simulink model "SP_OEL2"  (R2023b)
settings: Solver=ode23t  StartTime=0.0  StopTime=0.6  MaxStep=simulation.maxStepSize  RelTol=1e-3  AbsTol=1e-3
PostLoadFcn:
  | run('OCR_input.m');
  | run('OCR_settings.m');
InitFcn:
  | run('OCR_settings.m');
undefined symbols (not defined in the file or in its folder): relay1, relay2, source
libraries: ee_lib x14, fl_lib x8, eeGeneralControl x8, simulink x4, simulink_extras x4, nesl_utility x2
(part 2 of 2)

== system SP_OEL2/Relay1/Phase Protection Unit/Operating time /Lookup table  ==
  Current : Inport
  2-D Lookup Table : Lookup_n-D  BreakpointsForDimension1=currentPhase  BreakpointsForDimension2=tmsPhase  Table=topPhase  InterpMethod=Cubic spline  ExtrapMethod=Cubic spline  InternalRulePriority=Speed  RndMeth=Simplest
      settings: InputPortMap=u0,u1
  Constant12 : Constant  Value=phTimeSetting  VectorParams1D=off
  Constant14 : Constant  Value=topPhaseActual
  Constant15 : Constant  Value=relayCharacteristicPhase
  Demux2 : Demux  Outputs=3
  Max : MinMax  Function=max  Inputs=3
  Switch3 : Switch  Threshold=8  SaturateOnIntegerOverflow=off  InputSameDT=off
  Operating Time : Outport
  wires:
  Constant15/1 -> Switch3/2
  Current/1 -> Demux2/1
  Constant12/1 -> 2-D Lookup Table/2
  Demux2/2 -> Max/2
  Demux2/1 -> Max/1
  Constant14/1 -> Switch3/3
  2-D Lookup Table/1 -> Switch3/1
  Demux2/3 -> Max/3
  Switch3/1 -> Operating Time/1
  Max/1 -> 2-D Lookup Table/1

== system SP_OEL2/Relay2/Earth Protection Unit/Operating Time/Lookup table ==
  Current : Inport
  2-D Lookup Table1 : Lookup_n-D  BreakpointsForDimension1=currentEarth  BreakpointsForDimension2=tmsEarth  Table=topEarth  InterpMethod=Cubic spline  ExtrapMethod=Cubic spline  InternalRulePriority=Speed  RndMeth=Simplest
      settings: InputPortMap=u0,u1
  Constant13 : Constant  Value=ethTimeSetting
  Constant16 : Constant  Value=topEarthActual
  Constant17 : Constant  Value=relayCharacteristicEarth
  Switch4 : Switch  Threshold=8  SaturateOnIntegerOverflow=off  InputSameDT=off
  Oeprating Time : Outport
  wires:
  Current/1 -> 2-D Lookup Table1/1
  Constant17/1 -> Switch4/2
  2-D Lookup Table1/1 -> Switch4/1
  Constant16/1 -> Switch4/3
  Constant13/1 -> 2-D Lookup Table1/2
  Switch4/1 -> Oeprating Time/1

== system SP_OEL2/Relay2/Phase Protection Unit/Operating time /Lookup table  ==
  Current : Inport
  2-D Lookup Table : Lookup_n-D  BreakpointsForDimension1=currentPhase  BreakpointsForDimension2=tmsPhase  Table=topPhase  InterpMethod=Cubic spline  ExtrapMethod=Cubic spline  InternalRulePriority=Speed  RndMeth=Simplest
      settings: InputPortMap=u0,u1
  Constant12 : Constant  Value=phTimeSetting  VectorParams1D=off
  Constant14 : Constant  Value=topPhaseActual
  Constant15 : Constant  Value=relayCharacteristicPhase
  Demux2 : Demux  Outputs=3
  Max : MinMax  Function=max  Inputs=3
  Switch3 : Switch  Threshold=8  SaturateOnIntegerOverflow=off  InputSameDT=off
  Operating Time : Outport
  wires:
  Constant15/1 -> Switch3/2
  Current/1 -> Demux2/1
  Constant12/1 -> 2-D Lookup Table/2
  Demux2/2 -> Max/2
  Demux2/1 -> Max/1
  Constant14/1 -> Switch3/3
  2-D Lookup Table/1 -> Switch3/1
  Demux2/3 -> Max/3
  Switch3/1 -> Operating Time/1
  Max/1 -> 2-D Lookup Table/1

== matlab function SP_OEL2/Relay2/Earth Protection Unit/Operating Time/Standard Characteristics ==
  data: plugSetting input; operatingTime output; timeSetting input; relayCharacteristic input
function operatingTime = fcn(plugSetting,timeSetting,relayCharacteristic)
   if plugSetting>1             % Fault condition
    switch relayCharacteristic  % Selection of relay characteristic
        case 1                  % IEC Normal Inverse
          a=0.14;      
          b=0.02;
          c=0;
        case 2                  % IEC Very Inverse
           a=13.5;
           b=1;
           c=0;
        case 3                  % IEC Extremely Inverse
            a=80;
            b=2;
            c=0;
        case 4                  % IEC Moderately Inverse
            a=0.0515;
            b=0.02;
            c=0.114;
        case 5                  % IEEE Very Inverse
            a=19.61;
            b=2;
            c=0.491;
        case 6                  % IEEE Exteremely Inverse
            a=28.2;
            b=2;
            c=0.1217;
        otherwise               % Definite Time
            a=1;
            b=1;
            c=0;
            plugSetting=2;
    end               
         operatingTime=timeSetting*(a/(power(max(plugSetting),b)-1)+c);  % Calculate the oeprating time of the relay    
   else
       operatingTime=inf;  % Set relay operating time to infinite if there is no fault
   end
end

== matlab function SP_OEL2/Relay2/Phase Protection Unit/Operating time /MATLAB Function ==
  data: plugSetting input; operatingTime output; timeSetting input; relayCharacteristic input
function operatingTime = fcn(plugSetting,timeSetting,relayCharacteristic)
   if plugSetting(1)>1 || plugSetting(2)>1 || plugSetting(3)>1  % Fault condition
    switch relayCharacteristic  % Selection of relay characteristic
        case 1                  % IEC Normal Inverse
          a=0.14;      
          b=0.02;
          c=0;
        case 2                  % IEC Very Inverse
           a=13.5;
           b=1;
           c=0;
        case 3                  % IEC Extremely Inverse
            a=80;
            b=2;
            c=0;
        case 4                  % IEC Moderately Inverse
            a=0.0515;
            b=0.02;
            c=0.114;
        case 5                  % IEEE Very Inverse
            a=19.61;
            b=2;
            c=0.491;
        case 6                  % IEEE Exteremely Inverse
            a=28.2;
            b=2;
            c=0.1217;
        otherwise               % Definite Time
            a=1;
            b=1;
            c=0;
            plugSetting=ones(3,1)*2;
    end           
         
         operatingTime=timeSetting*(a/(power(max(plugSetting),b)-1)+c);  % Calculate oeprating time of the relay  
   else
         operatingTime=inf;  % Set relay operating time to infinite if there is no fault
   end
end

== matlab function SP_OEL2/Relay1/Earth Protection Unit/Operating Time/Standard Characteristics ==
  data: plugSetting input; operatingTime output; timeSetting input; relayCharacteristic input
function operatingTime = fcn(plugSetting,timeSetting,relayCharacteristic)
   if plugSetting>1             % Fault condition
    switch relayCharacteristic  % Selection of relay characteristic
        case 1                  % IEC Normal Inverse
          a=0.14;      
          b=0.02;
          c=0;
        case 2                  % IEC Very Inverse
           a=13.5;
           b=1;
           c=0;
        case 3                  % IEC Extremely Inverse
            a=80;
            b=2;
            c=0;
        case 4                  % IEC Moderately Inverse
            a=0.0515;
            b=0.02;
            c=0.114;
        case 5                  % IEEE Very Inverse
            a=19.61;
            b=2;
            c=0.491;
        case 6                  % IEEE Exteremely Inverse
            a=28.2;
            b=2;
            c=0.1217;
        otherwise               % Definite Time
            a=1;
            b=1;
            c=0;
            plugSetting=2;
    end               
         operatingTime=timeSetting*(a/(power(max(plugSetting),b)-1)+c);  % Calculate the oeprating time of the relay    
   else
       operatingTime=inf;  % Set relay operating time to infinite if there is no fault
   end
end

== matlab function SP_OEL2/Relay1/Phase Protection Unit/Operating time /MATLAB Function ==
  data: plugSetting input; operatingTime output; timeSetting input; relayCharacteristic input
function operatingTime = fcn(plugSetting,timeSetting,relayCharacteristic)
   if plugSetting(1)>1 || plugSetting(2)>1 || plugSetting(3)>1  % Fault condition
    switch relayCharacteristic  % Selection of relay characteristic
        case 1                  % IEC Normal Inverse
          a=0.14;      
          b=0.02;
          c=0;
        case 2                  % IEC Very Inverse
           a=13.5;
           b=1;
           c=0;
        case 3                  % IEC Extremely Inverse
            a=80;
            b=2;
            c=0;
        case 4                  % IEC Moderately Inverse
            a=0.0515;
            b=0.02;
            c=0.114;
        case 5                  % IEEE Very Inverse
            a=19.61;
            b=2;
            c=0.491;
        case 6                  % IEEE Exteremely Inverse
            a=28.2;
            b=2;
            c=0.1217;
        otherwise               % Definite Time
            a=1;
            b=1;
            c=0;
            plugSetting=ones(3,1)*2;
    end           
         
         operatingTime=timeSetting*(a/(power(max(plugSetting),b)-1)+c);  % Calculate oeprating time of the relay  
   else
         operatingTime=inf;  % Set relay operating time to infinite if there is no fault
   end
end
